simulink model "PrechargeModel"  (R2024a)
settings: Solver=ode23tb  StartTime=0.0  StopTime=10  MaxStep=1  MinStep=0.05  RelTol=1e-3
libraries: fl_lib x9, nesl_utility x9, ee_lib x2, eeSinusoidalMeasurementV2 x2, msbPllFoundation x2, batteryecm_lib x1, eeStairGenerator x1
settings Model: Creator=HP  LastModifiedBy=HP
settings SolverCC: InitialStep=0.1  SolverJacobianMethodControl=FullPerturbation
settings SimscapeCC: ExplicitSolverDiagnosticOptions=none

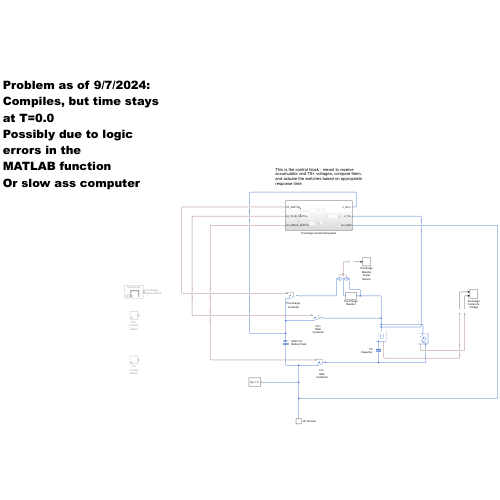
[thumbnail: Simulink's stored preview of the top-level diagram]
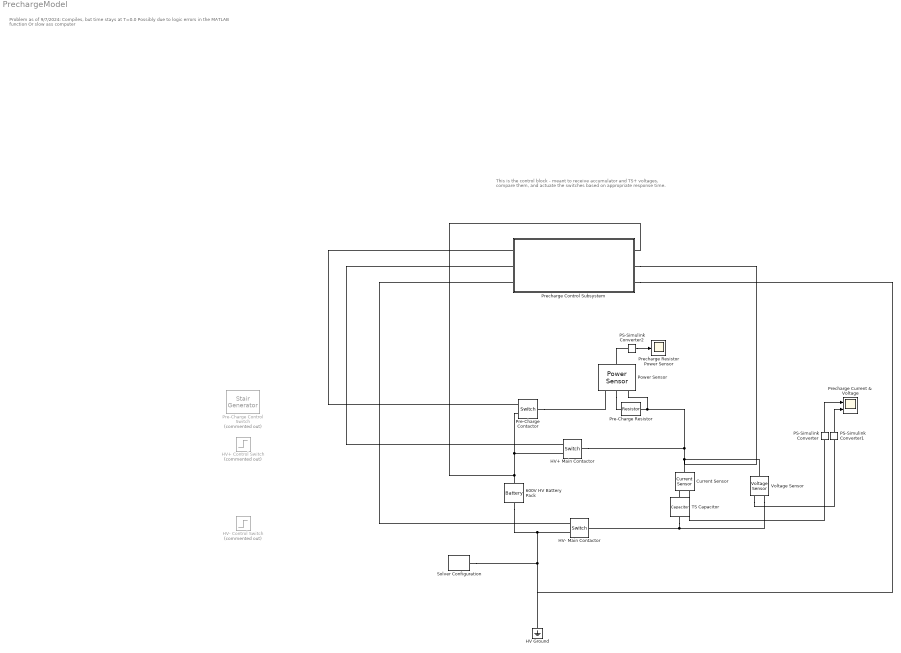
== system PrechargeModel ==
  note: Problem as of 9/7/2024:
      | Compiles, but time stays at T=0.0
      | Possibly due to logic errors in the
      | MATLAB function
      | Or slow ass computer
  note: This is the control block - meant to receive
      | accumulator and TS+ voltages, compare them,
      | and actuate the switches based on appropriate
      | response time.
  600V HV Battery Pack : batteryecm_lib/Battery  Vnom=600 V  prm_dir=simscape.enum.battery.prm_dir.disabled  R1_dis=2 Ohm  R1_ch=2 Ohm  R1=1 Ohm  prm_AH=simscape.enum.battery.prm_AH.infinite  AH=50 A*hr  V1=11.5 V  AH1=25 A*hr  prm_R2=simscape.enum.battery.prm_R2.disabled  R2=2000 Ohm  Tmeas=298.15 K  charge_measurement_port=simscape.enum.battery.enable.no  prm_dyn=simscape.enum.battery.prm_dyn.off  Rp1=0.005 Ohm  tau1=30 s  Rp2=0.005 Ohm  tau2=30 s  Rp3=0.005 Ohm  tau3=30 s  Rp4=0.005 Ohm  tau4=30 s  Rp5=0.005 Ohm  tau5=30 s  prm_fade=simscape.enum.battery.prm_fade.disabled  N_fade=100  AH_fade=45 A*hr  R1_fade=2.02 Ohm  R1_ch_fade=2.02 Ohm  V1_fade=10.35 V  prm_age=simscape.enum.battery.prm_age.disabled  prm_age_OCV=simscape.enum.battery.prm_age_OCV.OCV  OCV_age=0.9  SOC_age=60  Tmeas_age=298.15 K  delta_time_age_vec=[0] d  temperature_age_vec=[273] K  OCV_scaling_age=2.2134e6  OCV_offset_age=1.632e6  temp_exp_age=0.515833569 V  t_exp_age=0.75  Vnom_T2=12 V  R1_T2=2.2 Ohm  R1_T2_dis=2.2 Ohm  R1_T2_ch=2.2 Ohm  V1_T2=11.4 V  R2_T2=2200 Ohm  Rp1_T2=0.005 Ohm  tau1_T2=30 s  Rp2_T2=0.005 Ohm  tau2_T2=30 s  Rp3_T2=0.005 Ohm  tau3_T2=30 s  Rp4_T2=0.005 Ohm  tau4_T2=30 s  Rp5_T2=0.005 Ohm  tau5_T2=30 s  Tmeas2=273.15 K  thermal_port=simscape.enum.thermaleffects.omit  thermal_mass=30000 J/K  i_specify=off  i_priority=None  i=0 A  i_nominal_specify=off  i_nominal_value=1  i_nominal_unit=A  v_specify=off  v_priority=None  v=0 V  v_nominal_specify=off  v_nominal_value=1  v_nominal_unit=V  charge_specify=off  charge_priority=High  charge=50 A*hr  charge_nominal_specify=off  charge_nominal_value=1  charge_nominal_unit=A*hr  num_cycles_specify=off  num_cycles_priority=High  num_cycles=0  num_cycles_nominal_specify=off  num_cycles_nominal_value=1  num_cycles_nominal_unit=1  temperature_specify=off  temperature_priority=High  temperature=298.15 K  temperature_nominal_specify=off  temperature_nominal_value=1  temperature_nominal_unit=K
  Current Sensor : fl_lib/Electrical/Electrical Sensors/Current Sensor
  HV Ground : fl_lib/Electrical/Electrical Elements/Electrical Reference
  HV+ Main Contactor : fl_lib/Electrical/Electrical Elements/Switch  R_closed=0.01 Ohm  G_open=1e-8 1/Ohm  Threshold=0.5  i_specify=off  i_priority=None  i=0 A  i_nominal_specify=off  i_nominal_value=1  i_nominal_unit=A  v_specify=off  v_priority=None  v=0 V  v_nominal_specify=off  v_nominal_value=1  v_nominal_unit=V
  HV+ Control Switch : Step  Commented=on  Time=8  SampleTime=0
  HV- Control Switch : Step  Commented=on  Time=1.5  SampleTime=0
  HV- Main Contactor : fl_lib/Electrical/Electrical Elements/Switch  R_closed=0.01 Ohm  G_open=1e-8 1/Ohm  Threshold=0.5  i_specify=off  i_priority=None  i=0 A  i_nominal_specify=off  i_nominal_value=1  i_nominal_unit=A  v_specify=off  v_priority=None  v=0 V  v_nominal_specify=off  v_nominal_value=1  v_nominal_unit=V
  PS-Simulink Converter : nesl_utility/PS-Simulink Converter  PhysicalDomain=network_engine_domain  SubClassName=ps_output  LeftPortType=input  RightPortType=output  PseudoPeriodic=off  Frequencies=[]  VectorFormat=inherit  Unit=inherit  AffineConversion=off
  PS-Simulink Converter1 : nesl_utility/PS-Simulink Converter  PhysicalDomain=network_engine_domain  SubClassName=ps_output  LeftPortType=input  RightPortType=output  PseudoPeriodic=off  Frequencies=[]  VectorFormat=inherit  Unit=inherit  AffineConversion=off
  PS-Simulink Converter2 : nesl_utility/PS-Simulink Converter  PhysicalDomain=network_engine_domain  SubClassName=ps_output  LeftPortType=input  RightPortType=output  PseudoPeriodic=off  Frequencies=[]  VectorFormat=inherit  Unit=inherit  AffineConversion=off
  Power Sensor : ee_lib/Sensors & Transducers/Power Sensor  measurement_type=1  averaging_period=1e-4 s
  Pre-Charge Contactor : fl_lib/Electrical/Electrical Elements/Switch  R_closed=0.01 Ohm  G_open=1e-8 1/Ohm  Threshold=0.5  i_specify=off  i_priority=None  i=0 A  i_nominal_specify=off  i_nominal_value=1  i_nominal_unit=A  v_specify=off  v_priority=None  v=0 V  v_nominal_specify=off  v_nominal_value=1  v_nominal_unit=V
  Pre-Charge Control Switch : eeStairGenerator/Stair Generator  Commented=on  LabelModeActiveChoice=Continuous  TimeInput=[0 1 10]  AmplitudeInput=[0 1 0]  SampleTime=0  RepeatPattern=off  OutDataTypeStr=double
      settings: LibrarySourceBlock=ee_sl_lib/General Control/Stair Generator
  Pre-Charge Resistor : ee_lib/Passive/Resistor  R=780 Ohm  enable_R_tol=ee.enum.toleranceApplication.none  R_tol=5  tol_distribution=ee.enum.toleranceDistribution.uniform  nSigma=4  enable_operating_limits=ee.enum.enable.no  operating_limit_action=ee.enum.passive.reportOpLim.warn  power_rating=1 W  max_working_voltage=100 V  enable_faults=ee.enum.enable.no  fault_action=simscape.enum.assert.action.none  R_faulted=inf Ohm  fault_trigger=ee.enum.faults.faultTrigger.temporal  t_fault=1 s  max_permissible_current=1 A  t_fail_on_current=1 s  noise_mode=ee.enum.sources.noise.Disabled  Tdevice=25 degC  sample_time=1e-3 s  repeatability=ee.enum.ic.repeatability.notRepeatable  user_seed=0  auto_seed=3890346746  faulted_specify=off  faulted_priority=None  faulted=0  power_derating_T1=70 degC  power_derating_T2=155 degC  operating_temperature_range_vec=[-50, 150] degC  alpha=3.93e-3 1/K  Tmeas=25 degC  thermal_mass=100 J/K  temperature_specify=off  temperature_priority=High  temperature=298.15 K  temperature_nominal_specify=off  temperature_nominal_value=1  temperature_nominal_unit=K
  Precharge Current & Voltage : Scope  NumInputPorts=2
  Precharge Resistor Power Sensor : Scope
  Precharge Control Subsystem : Subsystem
  Solver Configuration : nesl_utility/Solver Configuration  PhysicalDomain=network_engine_domain  SubClassName=solver  LeftPortType=input  RightPortType=generic  Tones=[]  Harmonics=[]  SimulateNoise=off  Profile=off  UseLocalSampling=off  EnableSwitchedLinearOptims=on  FrequencyDomain=off  UseCCode=off  RelTol=0.001  AbsTol=0.001  MinStep=1e-09  ToWorkspace=off  RevertToSquareIcSolve=off  NumHomotopyIterations=100  PhasorMode=off  PhasorModeNumHarmonics=1  ConsistencySolver=NEWTON_XTOL_AFTER_FTOL  IndexReductionMethod=DerivativeReplacement  DoDC=off  ResidualTolerance=1e-09  ConsistencyTolSource=GLOBAL  ConsistencyAbsTol=0.001  ConsistencyRelTol=0.001  ConsistencyTolFactor=0.001  UseLocalSolver=on  LocalSolverChoice=NE_BACKWARD_EULER_ADVANCER  ResolveIndetEquations=on  FunctionEvalNumThread=1  LocalSolverSampleTime=0.001  DoFixedCost=on  MaxNonlinIter=3  MaxModeIter=2  ComputeImpulses=off  ImpulseIterations=2  LinearAlgebra=auto  LinearAlgebraNumThread=0  EquationFormulation=NE_TIME_EF  DelaysMemoryBudget=1024  AutomaticFiltering=on  FilteringTimeConstant=0.001  PartitionStorageMethod=AS_NEEDED  PartitionMemoryBudget=1024  PartitionMethod=ROBUST  MultibodyUseLocalSolver=off  MultibodyLocalSolverChoice=ODE1  MultibodyLocalSolverSampleTime=0.001
  TS Capacitor : fl_lib/Electrical/Electrical Elements/Capacitor  c=1.88 mF  r=1e-6 Ohm  g=0 1/Ohm  i_specify=off  i_priority=None  i=0 A  i_nominal_specify=off  i_nominal_value=1  i_nominal_unit=A  v_specify=off  v_priority=None  v=0 V  v_nominal_specify=off  v_nominal_value=1  v_nominal_unit=V  vc_specify=off  vc_priority=High  vc=0 V  vc_nominal_specify=off  vc_nominal_value=1  vc_nominal_unit=V
  Voltage Sensor : fl_lib/Electrical/Electrical Sensors/Voltage Sensor
  wires:
  PS-Simulink Converter/1 -> Precharge Current & Voltage/1
  PS-Simulink Converter1/1 -> Precharge Current & Voltage/2
  PS-Simulink Converter2/1 -> Precharge Resistor Power Sensor/1
  connections:
  600V HV Battery Pack/LConn1 -- Precharge Control Subsystem/RConn1 -- HV+ Main Contactor/RConn2 -- Pre-Charge Contactor/RConn2
  Pre-Charge Contactor/LConn1 -- Power Sensor/LConn1
  Pre-Charge Resistor/RConn1 -- Power Sensor/LConn3 -- Precharge Control Subsystem/RConn2 -- Current Sensor/LConn1 -- Voltage Sensor/LConn1 -- HV+ Main Contactor/LConn1
  Current Sensor/RConn2 -- TS Capacitor/LConn1
  600V HV Battery Pack/RConn1 -- HV Ground/LConn1 -- Precharge Control Subsystem/RConn3 -- Solver Configuration/RConn1 -- HV- Main Contactor/RConn2
  TS Capacitor/RConn1 -- HV- Main Contactor/LConn1 -- Voltage Sensor/RConn2
  Current Sensor/RConn1 -- PS-Simulink Converter/LConn1
  Voltage Sensor/RConn1 -- PS-Simulink Converter1/LConn1
  Power Sensor/LConn2 -- Pre-Charge Resistor/LConn1
  Power Sensor/RConn1 -- PS-Simulink Converter2/LConn1
  Precharge Control Subsystem/LConn1 -- Pre-Charge Contactor/RConn1
  Precharge Control Subsystem/LConn2 -- HV+ Main Contactor/RConn1
  Precharge Control Subsystem/LConn3 -- HV- Main Contactor/RConn1

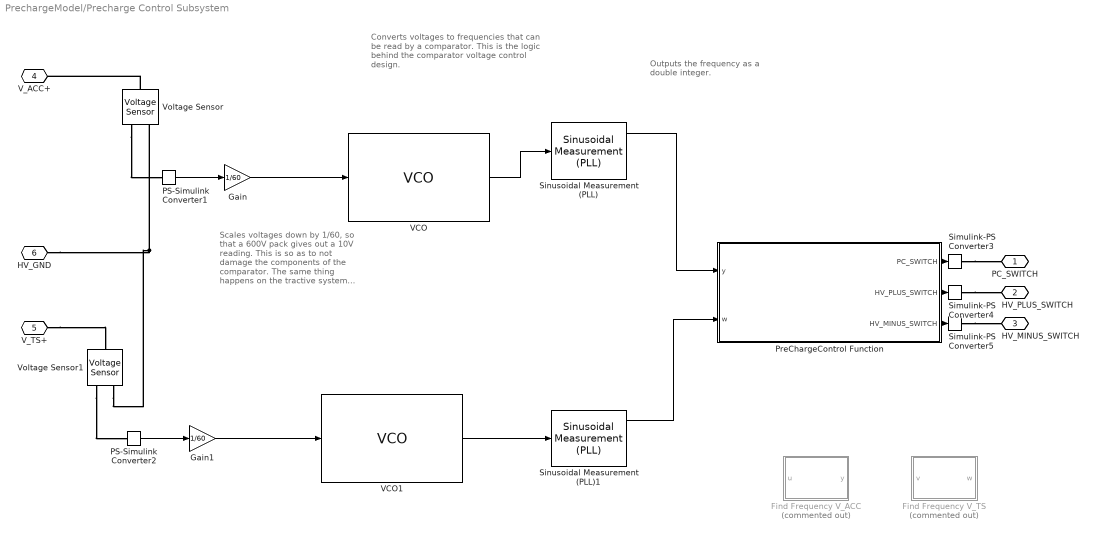
== system PrechargeModel/Precharge Control Subsystem ==
  note: Outputs the frequency
      | as a double integer.
  note: Converts voltages to frequencies
      | that can be read by a comparator.
      | This is the logic behind the comparator
      | voltage control design.
  note: Scales voltages down
      | by 1/60, so that a 600V
      | pack gives out a 10V reading.
      | This is so as to not damage the
      | components of the comparator.
      | The same thing happens on
      | the tractive system side.
  Find Frequency V_ACC : MATLAB Function  Commented=on  TreatAsAtomicUnit=on
  Find Frequency V_TS : MATLAB Function  Commented=on  TreatAsAtomicUnit=on
  Gain : Gain  Gain=1/60
  Gain1 : Gain  Gain=1/60
  PS-Simulink Converter1 : nesl_utility/PS-Simulink Converter  PhysicalDomain=network_engine_domain  SubClassName=ps_output  LeftPortType=input  RightPortType=output  PseudoPeriodic=off  Frequencies=[]  VectorFormat=inherit  Unit=inherit  AffineConversion=off
  PS-Simulink Converter2 : nesl_utility/PS-Simulink Converter  PhysicalDomain=network_engine_domain  SubClassName=ps_output  LeftPortType=input  RightPortType=output  PseudoPeriodic=off  Frequencies=[]  VectorFormat=inherit  Unit=inherit  AffineConversion=off
  PreChargeControl Function : MATLAB Function  TreatAsAtomicUnit=on
  Simulink-PS Converter3 : nesl_utility/Simulink-PS Converter  PhysicalDomain=network_engine_domain  SubClassName=ps_input  LeftPortType=input  RightPortType=output  PseudoPeriodic=off  Frequencies=[]  NoiseDistribution=none  NoiseParameters=[]  Unit=1  AffineConversion=off  FilteringAndDerivatives=provide  SimscapeFilterOrder=1  InputFilterTimeConstant=0.001  UdotUserProvided=0
  Simulink-PS Converter4 : nesl_utility/Simulink-PS Converter  PhysicalDomain=network_engine_domain  SubClassName=ps_input  LeftPortType=input  RightPortType=output  PseudoPeriodic=off  Frequencies=[]  NoiseDistribution=none  NoiseParameters=[]  Unit=1  AffineConversion=off  FilteringAndDerivatives=provide  SimscapeFilterOrder=1  InputFilterTimeConstant=0.001  UdotUserProvided=0
  Simulink-PS Converter5 : nesl_utility/Simulink-PS Converter  PhysicalDomain=network_engine_domain  SubClassName=ps_input  LeftPortType=input  RightPortType=output  PseudoPeriodic=off  Frequencies=[]  NoiseDistribution=none  NoiseParameters=[]  Unit=1  AffineConversion=off  FilteringAndDerivatives=provide  SimscapeFilterOrder=1  InputFilterTimeConstant=0.001  UdotUserProvided=0
  Sinusoidal Measurement (PLL) : eeSinusoidalMeasurementV2/Sinusoidal Measurement (PLL)  Ki_PD=1000  Kp_LF=400  Ki_LF=20000  F0=60  Theta0=0  Mag0=1  Ts=-1
      settings: LibrarySourceBlock=|
      | ee_sl_lib/Measurements/Sinusoidal Measurement
      | (PLL)
  Sinusoidal Measurement (PLL)1 : eeSinusoidalMeasurementV2/Sinusoidal Measurement (PLL)  Ki_PD=1000  Kp_LF=400  Ki_LF=20000  F0=60  Theta0=0  Mag0=1  Ts=-1
      settings: LibrarySourceBlock=|
      | ee_sl_lib/Measurements/Sinusoidal Measurement
      | (PLL)
  VCO : msbPllFoundation/VCO  SpecifyUsing=Voltage sensitivity  Kvco=100  Fo=2.5e9  ControlVoltage=[-5 0 5]  OutputFrequency=[2e9 2.5e9 3e9]  Amplitude=1  ExtraBuffer=off  NBuffer=1000  AddPhaseNoise=off  Foffset=[10e3 100e3 1e6 3e6 10e6]  PhaseNoise=[-77 -108 -134 -145 -154]  MaxKvco=100
  VCO1 : msbPllFoundation/VCO  SpecifyUsing=Voltage sensitivity  Kvco=100  Fo=2.5e9  ControlVoltage=[-5 0 5]  OutputFrequency=[2e9 2.5e9 3e9]  Amplitude=1  ExtraBuffer=off  NBuffer=1000  AddPhaseNoise=off  Foffset=[10e3 100e3 1e6 3e6 10e6]  PhaseNoise=[-77 -108 -134 -145 -154]  MaxKvco=100
  Voltage Sensor : fl_lib/Electrical/Electrical Sensors/Voltage Sensor
  Voltage Sensor1 : fl_lib/Electrical/Electrical Sensors/Voltage Sensor
  HV_PLUS_SWITCH : PMIOPort  Port=2  Side=Left
  HV_MINUS_SWITCH : PMIOPort  Port=3  Side=Left
  V_ACC+ : PMIOPort  Port=4  Side=Right
  V_TS+ : PMIOPort  Port=5  Side=Right
  HV_GND : PMIOPort  Port=6  Side=Right
  PC_SWITCH : PMIOPort  Side=Left
  wires:
  Gain/1 -> VCO/1
  VCO/1 -> Sinusoidal Measurement (PLL)/1
  PS-Simulink Converter1/1 -> Gain/1
  VCO1/1 -> Sinusoidal Measurement (PLL)1/1
  PS-Simulink Converter2/1 -> Gain1/1
  Gain1/1 -> VCO1/1
  PreChargeControl Function/1(PC_SWITCH) -> Simulink-PS Converter3/1
  PreChargeControl Function/2(HV_PLUS_SWITCH) -> Simulink-PS Converter4/1
  PreChargeControl Function/3(HV_MINUS_SWITCH) -> Simulink-PS Converter5/1
  Sinusoidal Measurement (PLL)/1 -> PreChargeControl Function/1(y)
  Sinusoidal Measurement (PLL)1/1 -> PreChargeControl Function/2(w)
  connections:
  Simulink-PS Converter3/RConn1 -- PC_SWITCH/RConn1
  Simulink-PS Converter5/RConn1 -- HV_MINUS_SWITCH/RConn1
  Simulink-PS Converter4/RConn1 -- HV_PLUS_SWITCH/RConn1
  Voltage Sensor/RConn1 -- PS-Simulink Converter1/LConn1
  Voltage Sensor/LConn1 -- V_ACC+/RConn1
  V_TS+/RConn1 -- Voltage Sensor1/LConn1
  Voltage Sensor1/RConn1 -- PS-Simulink Converter2/LConn1
  HV_GND/RConn1 -- Voltage Sensor1/RConn2 -- Voltage Sensor/RConn2

== matlab function PrechargeModel/Precharge Control Subsystem/Find Frequency V_TS ==
  data: v input; w output
function w = FindFrequency(v)
    % FindFrequency - Estimate the frequency of a sinusoidal signal.
    % Input:
    %   v - Vector of the sinusoidal signal values
    % Output:
    %   w - Estimated frequency of the sinusoidal signal in Hz

    % Ensure the input is a row vector
    v = v(:)';

    % Time vector assuming a sampling frequency
    fs = 1000; % Sampling frequency in Hz (adjust as needed)
    t = (0:length(v)-1) / fs;

    % Compute the derivative of the signal
    dv = diff(v);

    % Find zero-crossings of the derivative
    zeroCrossings = find((dv(1:end-1) >= 0 & dv(2:end) < 0) | (dv(1:end-1) <= 0 & dv(2:end) > 0));

    % Ensure there are at least two zero-crossings to compute the period
    if length(zeroCrossings) < 2
        error('Not enough zero-crossings detected to estimate frequency.');
    end

    % Calculate the time intervals between zero-crossings
    zeroCrossingTimes = t(zeroCrossings);
    timeIntervals = diff(zeroCrossingTimes);

    % Compute the average period
    avgPeriod = mean(timeIntervals);

    % Compute the frequency
    w = 1 / avgPeriod;
end

== matlab function PrechargeModel/Precharge Control Subsystem/Find Frequency V_ACC ==
  data: u input; y output
function y = FindFrequency(u)
    % FindFrequency - Estimate the frequency of a sinusoidal signal.
    % Input:
    %   u - Vector of the sinusoidal signal values
    % Output:
    %   y - Estimated frequency of the sinusoidal signal in Hz

    % Ensure the input is a row vector
    u = u(:)';

    % Time vector assuming a sampling frequency
    fs = 1000; % Sampling frequency in Hz (adjust as needed)
    t = (0:length(u)-1) / fs;

    % Compute the derivative of the signal
    du = diff(u);

    % Find zero-crossings of the derivative
    zeroCrossings = find((du(1:end-1) >= 0 & du(2:end) < 0) | (du(1:end-1) <= 0 & du(2:end) > 0));

    % Ensure there are at least two zero-crossings to compute the period
    if length(zeroCrossings) < 2
        error('Not enough zero-crossings detected to estimate frequency.');
    end

    % Calculate the time intervals between zero-crossings
    zeroCrossingTimes = t(zeroCrossings);
    timeIntervals = diff(zeroCrossingTimes);

    % Compute the average period
    avgPeriod = mean(timeIntervals);

    % Compute the frequency
    y = 1 / avgPeriod;
end

== matlab function PrechargeModel/Precharge Control Subsystem/PreChargeControl Function ==
  data: y input; PC_SWITCH output; w input; HV_PLUS_SWITCH output; HV_MINUS_SWITCH output
function [PC_SWITCH, HV_PLUS_SWITCH, HV_MINUS_SWITCH] = PreChargeControl(y, w)
    %Function Algorithm: 
    %1) Measure the voltage-based frequencies across the accumulator and
    %TS, (y,w) respectively
    %Send 1 to precharge and MINUS contactor switches
    %2) When TS voltage is about 99% equal to ACC voltage (after 5TAU),
    %CHECK if the time it took for this to happen is within 4TAU-7TAU
    %This is to make sure any open/short circuits are prevented
    %If all is clear, output 1 to the MAIN contactor switch
    %0 to precharge contactor to open it once TS is fully charged



    %Changed based on plant model
    R = 780; % Resistance in ohms
    C = 0.188; % Capacitance in farads

    % Precharge time limits
    minTime = 4 * R * C;
    maxTime = 7 * R * C;

    % Initialize control signals
    PC_SWITCH = 0;
    HV_PLUS_SWITCH = 0;
    HV_MINUS_SWITCH = 0;

    % Start precharge sequence
    PC_SWITCH = 1;
    HV_MINUS_SWITCH = 1;

    % Start timer
    timerStart = tic;
    timerValue = 0; % Initialize timerValue to ensure it's defined

    % Initialize loop variables
    maxIterations = 1000; % Set a maximum number of iterations
    iterationCount = 0;

    % Wait for frequency condition or timeout
    while iterationCount < maxIterations
        % Update timer value
        timerValue = toc(timerStart);
        iterationCount = iterationCount + 1;

        % Compare frequencies
        if abs(w - y) / y <= 0.05
            break;
        end

        % Check timer for timeout condition
        if timerValue > maxTime
            break;
        end
    end

    % Check if timer is within acceptable range
    if timerValue < minTime || timerValue > maxTime
        PC_SWITCH = 0; % Turn off PC switch
    else
        HV_PLUS_SWITCH = 1; % Turn on HV Plus switch
    end

    % Reset HV_MINUS_SWITCH (assuming it should be turned off after the process)
    % HV_MINUS_SWITCH = 0;
end
